simulink model "library_test"  (R2024b)
settings: Solver=ode1  StartTime=0.0  StopTime=100  FixedStep=1/500.  RelTol=1e-3
libraries: sdu_controllers x2
settings Model: Creator=eld  LastModifiedBy=eld

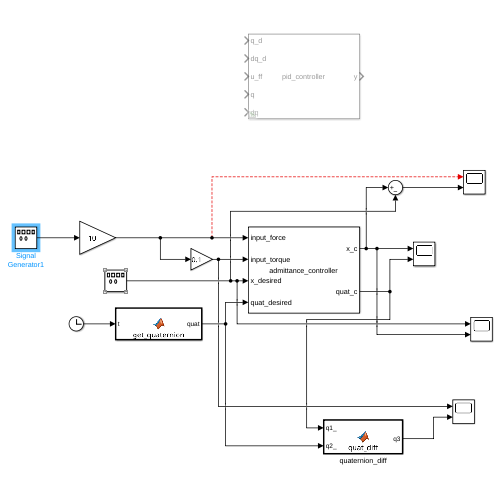
[thumbnail: Simulink's stored preview of the top-level diagram]
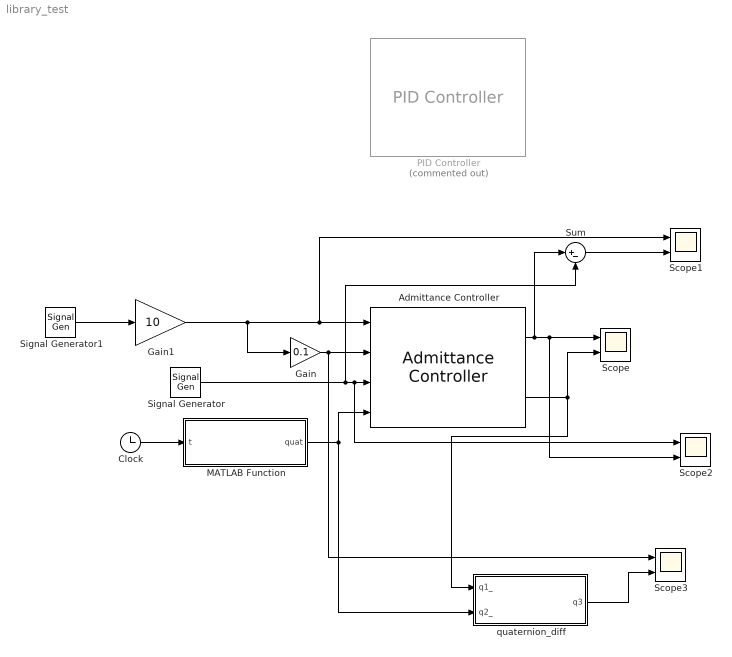
== system library_test ==
  Admittance Controller : sdu_controllers/Admittance Controller  Mp=eye( 3 ) * 22.5  Kp="eye( 3 ) *  55"  Dp=eye(3) * 70  Mo=eye( 3 ) * 0.25  Ko=eye( 3 ) * 10  Do=eye( 3 ) * 3  sample_time=1 / 500.  SimulateUsing=Interpreted execution
  Clock : Clock
  Gain : Gain  Gain=0.1
  Gain1 : Gain  Gain=10
  MATLAB Function : MATLAB Function  TreatAsAtomicUnit=on
  PID Controller : sdu_controllers/PID Controller  Commented=on  Kp=100.0  Ki=0.0  Kd=2 * sqrt( 100.0 )  N=1  num_states=6  sample_time=1 / 500.  SimulateUsing=Interpreted execution
  Scope{,1..3} (4 alike) : Scope  NumInputPorts=2
  Signal Generator : SignalGenerator  Amplitude=[1, 2, 3]  Units=rad/sec
  Signal Generator1 : SignalGenerator  WaveForm=square  Amplitude=[1, 2, 3]  Frequency=[1.0,1.1,1.2] * 0.5  Units=rad/sec
  Sum : Sum  Inputs=|+-
  quaternion_diff : MATLAB Function  TreatAsAtomicUnit=on
  wires:
  Signal Generator/1 -> Sum/2, Scope2/1, Admittance Controller/3
  MATLAB Function/1(quat) -> quaternion_diff/2(q2_), Admittance Controller/4
  Clock/1 -> MATLAB Function/1(t)
  Signal Generator1/1 -> Gain1/1
  Gain/1 -> Admittance Controller/2, Scope3/1
  Admittance Controller/1 -> Sum/1, Scope2/2, Scope/1
  Admittance Controller/2 -> Scope/2, quaternion_diff/1(q1_)
  Gain1/1 -> Gain/1, Scope1/1, Admittance Controller/1
  Sum/1 -> Scope1/2
  quaternion_diff/1(q3) -> Scope3/2

== matlab function library_test/MATLAB Function ==
  data: t input; quat output
function quat = get_quaternion(t)

q1 = quaternion(1, 0, 0, 0);
q1 = q1 / norm(q1);

%
q2 = quaternion(2, 3, 4, 5);
q2 = q2 / norm(q2);

qout = slerp(q1, q2, t/100);

quat = compact(qout);

== matlab function library_test/quaternion_diff ==
  data: q1_ input; q3 output; q2_ input
function q3 = quat_diff(q1_, q2_)

q1 = quaternion(q1_);
q2 = quaternion(q2_);

q3 = compact(q1 - q2);
